simulink model "third_task"  (R2022a)
settings: Solver=VariableStepAuto  StartTime=0.0  StopTime=0.017  RelTol=1e-3
libraries: commrandsrc3 x1, commutil2 x1
settings Model: Creator=Admin  LastModifiedBy=Admin

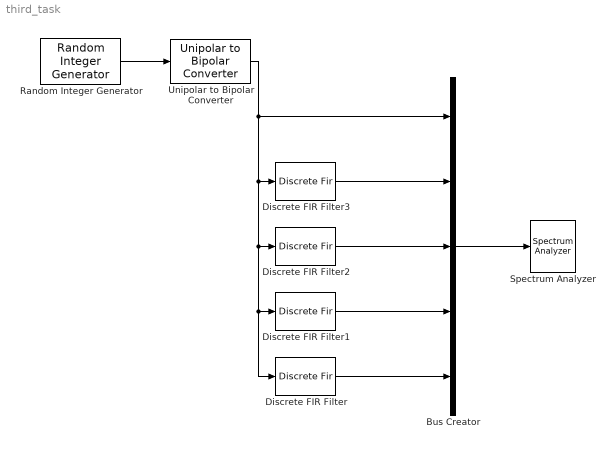
== system third_task ==
  Bus Creator : BusCreator  Inputs=5
  Discrete FIR Filter : DiscreteFir
  Discrete FIR Filter1 : DiscreteFir
  Discrete FIR Filter2 : DiscreteFir
  Discrete FIR Filter3 : DiscreteFir  InitialStates=0.7
  Random Integer Generator : commrandsrc3/Random Integer Generator  SetSize=2  SeedSource=Parameter  Seed=500  SampleTime=1/270000  SamplesPerFrame=1  OutputDataType=double  SimulateUsing=Interpreted execution
  Spectrum Analyzer : SpectrumAnalyzer
  Unipolar to Bipolar Converter : commutil2/Unipolar to Bipolar Converter  M=2  polarity=Positive  dataType=Inherit via internal rule
  wires:
  Random Integer Generator/1 -> Unipolar to Bipolar Converter/1
  Discrete FIR Filter3/1 -> Bus Creator/2
  Discrete FIR Filter2/1 -> Bus Creator/3
  Discrete FIR Filter1/1 -> Bus Creator/4
  Discrete FIR Filter/1 -> Bus Creator/5
  Bus Creator/1 -> Spectrum Analyzer/1
  Unipolar to Bipolar Converter/1 -> Bus Creator/1, Discrete FIR Filter/1, Discrete FIR Filter1/1, Discrete FIR Filter2/1, Discrete FIR Filter3/1
